simulink model "target_model"  (R2019a)
settings: Solver=FixedStepDiscrete  StartTime=0.0  StopTime=inf  RelTol=1e-3  EnableMultiTasking=on
PreLoadFcn:
  | load('visionhdlLaneDetectionInit.mat');
  | 
  | %Birds-Eye View Parameters:
  | T_unreal = [-0.346719845290643,-3.45626583672944e-16,-2.42608110520569e-19;-1.76272742794994,-2.62399506819665,-0.00185184300876343;1283.14845282490,1569.57420684550,1];
  | shiftleft = single([-5,-5,-5,-5,-5,-5,-5,-5,-5,-5,   -5,-4,-2,-2,-2,-2,0,0,0,1,    1,2,3,4,5,6,7,10,11,13,     15,17,20,22,26,30,33,38,42,46]);
  | shiftright = single([-20,-20,-20,-20,-20,-20,-20,-20,-20,-20,    -20,-20,-20,-21,-22,-23,-24,-24,-24,-25,    -26,-27,-28,-29,-30,-32,-33,-35,-37,-39,    -41,-45,-46,-50,-53,-57,-61,-67,-72,-78]);
StartFcn:
  | warning('off','Coder:MATLAB:polyfit_RepeatedPointsOrRescale');
  | warning('off','Coder:MATLAB:rankDeficientMatrix');
StopFcn:
  | warning('on','Coder:MATLAB:polyfit_RepeatedPointsOrRescale');
  | warning('on','Coder:MATLAB:rankDeficientMatrix');
undefined symbols (not defined in the file): FPGALaneDetection, IO333, LaneDetectionFPGA_final, msgfpgachecks, SFP
libraries: speedgoatlib_hdlCoder_IO333 x8, xpcutilitieslib x3, visiongeotforms x3, simulink x2, visiontextngfix x2, xpcvideoutillib x2, speedgoatlib_hdlCoder_IO333_vision x1, xpcrtudplib x1
Description:
  | Lane Detection
  | Detect lanes from streaming video.
settings Model: Creator=The MathWorks, Inc.  LastModifiedBy=timo.straessle
settings SolverCC: ConcurrentTasks=on  AutoInsertRateTranBlk=on
settings DataIOCC: SaveFormat=StructureWithTime  SaveOutput=off  SaveTime=off  ReturnWorkspaceOutputs=off
settings OptimizationCC: BlockReduction=off  ConditionallyExecuteInputs=off  DefaultParameterBehavior=Inlined  OptimizeBlockIOStorage=off  BufferReuse=off  GlobalBufferReuse=off  ExpressionFolding=off  LocalBlockOutputs=off  EfficientMapNaN2IntZero=off  OptimizeDataStoreBuffers=off  BusAssignmentInplaceUpdate=off
settings DebuggingCC: AlgebraicLoopMsg=error  SingleTaskRateTransMsg=error  ParameterPrecisionLossMsg=none  StrictBusMsg=ErrorOnBusTreatedAsVector  ArithmeticOperatorsInVariantConditions=warning
settings HardwareCC: ProdBitPerPointer=32  ProdBitPerSizeT=32  ProdBitPerPtrDiffT=32  ProdLargestAtomicFloat=None  ProdWordSize=32  ProdLongLongMode=on  ProdHWDeviceType=Generic->32-bit x86 compatible  TargetBitPerPointer=64  TargetBitPerSizeT=64  TargetBitPerPtrDiffT=64  TargetLongLongMode=on  TargetIntDivRoundTo=Zero  TargetEndianess=LittleEndian  TargetWordSize=64  TargetHWDeviceType=MATLAB Host
settings SFSimCC: SimUseLocalCustomCode=off
settings RTWCC: SystemTargetFile=slrt.tlc  TLCOptions=-axpcCPUClockPoll=0  TemplateMakefile=slrt_default_tmf  Description=Simulink Real-Time  CodeExecutionProfiling=on  RTWCompilerOptimization=on
settings CodeAppCC: MaxIdLength=128
settings SimulinkRealTimeCC: SupportVariableSizeSignals=on  PreserveStateflowLocalDataDimensions=off  RL32LogTETModifier=off  xPCisModelTimeout=off  xPCModelTimeoutSecs=60  xPCConcurrentTasks=on
settings ConfigComp: CovMetricSettings=dsw  CovHtmlReporting=on  CovSaveCumulativeToWorkspaceVar=on  CovSaveSingleToWorkspaceVar=on  CovShowResultsExplorer=off  CovExternalEMLEnable=off

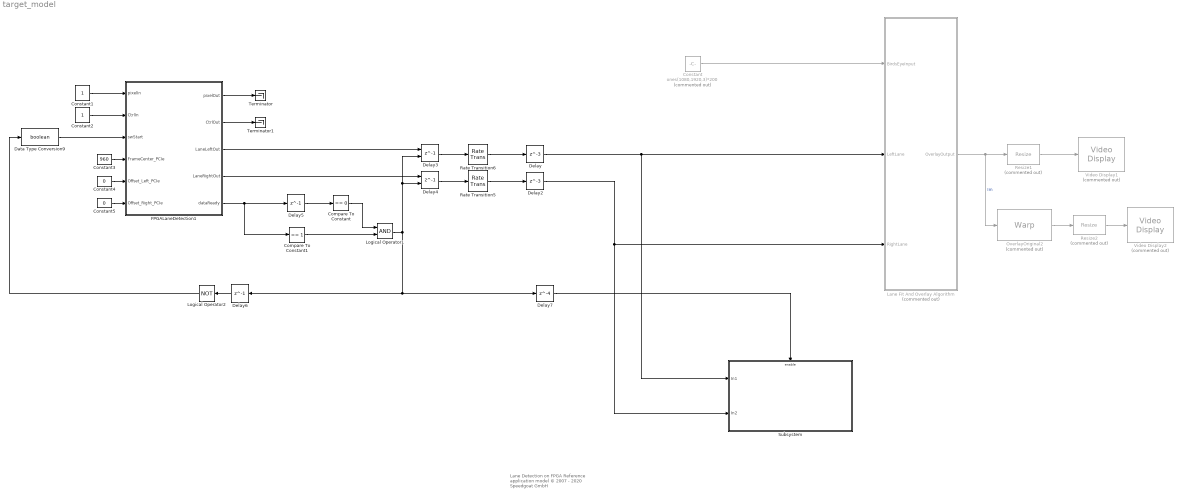
== system target_model ==
  note: Lane Detection on FPGA
      |
      | Reference application model
      | © 2007 - 2020 Speedgoat GmbH
  Compare To Constant : simulink/Logic and Bit Operations/Compare To Constant  relop===  const=0  OutDataTypeStr=boolean
  Compare To Constant1 : simulink/Logic and Bit Operations/Compare To Constant  relop===  const=1  OutDataTypeStr=boolean
  Constant : Constant  Commented=on  Value=ones(1080,1920,3)*200  OutDataTypeStr=uint8
  Constant1 : Constant
  Constant2 : Constant
  Constant3 : Constant  Value=960  OutDataTypeStr=fixdt(1,12,2^0,0)  SampleTime=-1
  Constant4 : Constant  Value=0  OutDataTypeStr=Inherit: Inherit via back propagation  SampleTime=-1
  Constant5 : Constant  Value=0  OutDataTypeStr=Inherit: Inherit via back propagation  SampleTime=-1
  Data Type Conversion9 : DataTypeConversion  OutDataTypeStr=boolean
  Delay : Delay  DelayLength=3
  Delay2 : Delay  DelayLength=3
  Delay3 : Delay  DelayLength=1  ShowEnablePort=on
      settings: InputPortMap=u0,e6
  Delay4 : Delay  DelayLength=1  ShowEnablePort=on
      settings: InputPortMap=u0,e6
  Delay5 : Delay  DelayLength=1
  Delay6 : Delay  DelayLength=1
  Delay7 : Delay  DelayLength=4
  FPGALaneDetection1 : Subsystem  InitFcn=msgfpgachecks;  mask(Speedgoat IO333-325k-SFP Interface Block){deviceIdx=0, slot=-1, ts=-1}
      mask prompts: deviceIdx "Device index:"; slot "PCI slot (-1: autosearch):"; ts "Sample time:"
      mask help: Simulink Real-Time Interface Block for Speedgoat IO333-325k-SFP.
      mask init:
      | mfpgaparameters;
      | TS = sg_hdlCoder_timestamp2DUTmask();
      mask Help: eval('speedgoatdoc_hdlc')
      mask Display: disp(sprintf('Speedgoat IO333-325k-SFP\nFPGA I/O Module\n\nTimestamp\n%s\n\nReference Design\nVersion 1.1\n\nMatlab R2019a\n\nPCIe Link Width: X4\nAurora Line Rate: 3.125\nAurora Byteswap: true\n', TS))
  Lane Fit And Overlay Algorithm : Subsystem  Commented=on
  Logical Operator1 : Logic  AllPortsSameDT=off  OutDataTypeStr=boolean
  Logical Operator2 : Logic  Operator=NOT  AllPortsSameDT=off  OutDataTypeStr=boolean
  OverlayOriginal2 : visiongeotforms/Warp  Commented=on  TransformMatrixSource=Custom  TransformMatrix=inv(T_unreal)  InterpolationMethod=Bilinear  BackgroundFillValue=0  OutputImagePositionSource=Custom  OutputImagePosition=[ 1, 1, 1920, 1080 ]  ROIInputPort=off  ROIValidityOutputPort=off  SimulateUsing=Code generation
      settings: SourceProductName=Computer Vision Toolbox  SourceProductBaseCode=VP
  Rate Transition5 : RateTransition  Deterministic=off  OutPortSampleTime=1/60
  Rate Transition6 : RateTransition  Deterministic=off  OutPortSampleTime=1/60
  Resize1 : visiongeotforms/Resize  Commented=on  specify=Output size as a percentage of input size  rfactor=[25 25]  outCols=25  outRows=25  outRowsCols=[25 35]  interp_method=Bilinear  antialias=on  useROI=off  roiFlag=off  roundingMode=Nearest  overflowMode=on  prodOutputMode=Binary point scaling  prodOutputWordLength=32  prodOutputFracLength=10  prodOutputSlope=2^-10  accumSlope=2^-10  outputSlope=2^-10
      settings: SourceProductName=Computer Vision Toolbox  SourceProductBaseCode=VP
  Resize2 : visiongeotforms/Resize  Commented=on  specify=Output size as a percentage of input size  rfactor=[25 25]  outCols=25  outRows=25  outRowsCols=[25 35]  interp_method=Bilinear  antialias=on  useROI=off  roiFlag=off  roundingMode=Nearest  overflowMode=on  prodOutputMode=Binary point scaling  prodOutputWordLength=32  prodOutputFracLength=10  prodOutputSlope=2^-10  accumSlope=2^-10  outputSlope=2^-10
      settings: SourceProductName=Computer Vision Toolbox  SourceProductBaseCode=VP
  Subsystem : Subsystem
  Terminator : Terminator
  Terminator1 : Terminator
  Video Display1 : xpcvideoutillib/Video Display  Commented=on  imagesignal=Single multidimensional signal  colorspace=RGB  vindex=1  showpreview=on
      settings: SourceProductName=Simulink Real-Time  SourceProductBaseCode=XP
  Video Display2 : xpcvideoutillib/Video Display  Commented=on  imagesignal=Single multidimensional signal  colorspace=RGB  vindex=2  showpreview=on
      settings: SourceProductName=Simulink Real-Time  SourceProductBaseCode=XP
  wires:
  Constant5/1 -> FPGALaneDetection1/6(Offset_Right_PCIe)
  Constant4/1 -> FPGALaneDetection1/5(Offset_Left_PCIe)
  Constant3/1 -> FPGALaneDetection1/4(FrameCenter_PCIe)
  Delay7/1 -> Subsystem/Enable
  Rate Transition6/1 -> Delay/1
  OverlayOriginal2/1 -> Resize2/1
  Delay2/1 -> Subsystem/2(In2), Lane Fit And Overlay Algorithm/3(RightLane)
  Delay4/1 -> Rate Transition5/1
  Rate Transition5/1 -> Delay2/1
  Compare To Constant1/1 -> Logical Operator1/2
  FPGALaneDetection1/5(dataReady) -> Compare To Constant1/1, Delay5/1
  Compare To Constant/1 -> Logical Operator1/1
  Logical Operator1/1 -> Delay7/1, Delay6/1, Delay4/2, Delay3/2
  Constant1/1 -> FPGALaneDetection1/1(pixelIn)
  Constant2/1 -> FPGALaneDetection1/2(CtrlIn)
  Resize2/1 -> Video Display2/1
  FPGALaneDetection1/2(CtrlOut) -> Terminator1/1
  FPGALaneDetection1/1(pixelOut) -> Terminator/1
  Delay5/1 -> Compare To Constant/1
  Lane Fit And Overlay Algorithm/1(OverlayOutput) -> Resize1/1, OverlayOriginal2/1  "Im"
  Delay3/1 -> Rate Transition6/1
  Logical Operator2/1 -> Data Type Conversion9/1
  FPGALaneDetection1/3(LaneLeftOut) -> Delay3/1
  Resize1/1 -> Video Display1/1
  Delay6/1 -> Logical Operator2/1
  FPGALaneDetection1/4(LaneRightOut) -> Delay4/1
  Constant/1 -> Lane Fit And Overlay Algorithm/1(BirdsEyeInput)
  Data Type Conversion9/1 -> FPGALaneDetection1/3(swStart)
  Delay/1 -> Subsystem/1(In1), Lane Fit And Overlay Algorithm/2(LeftLane)

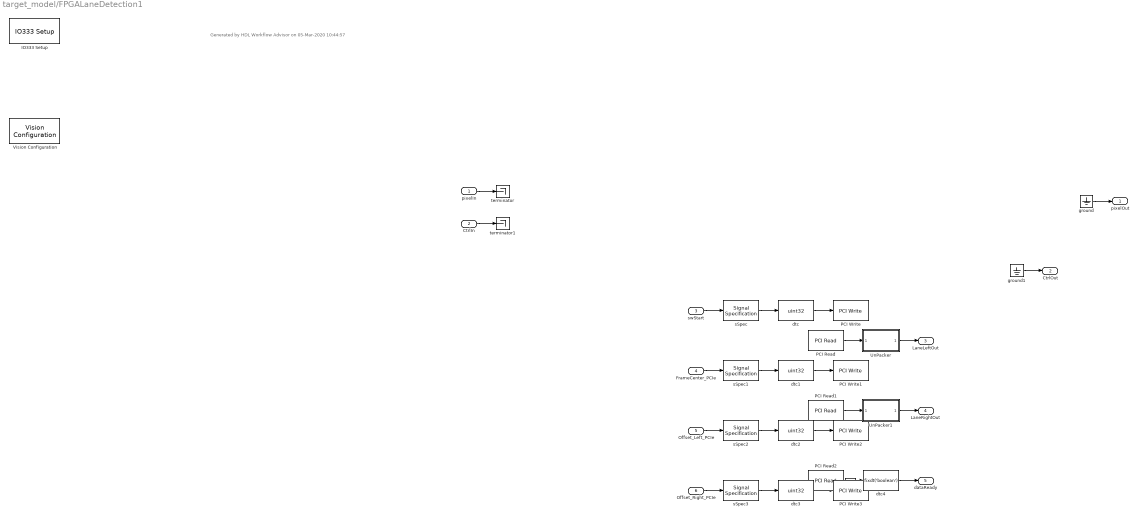
== system target_model/FPGALaneDetection1 ==
  note: Generated by HDL Workflow Advisor on 05-Mar-2020 10:44:57
  pixelIn : Inport
  CtrlIn : Inport  Port=2
  swStart : Inport  Port=3
  FrameCenter_PCIe : Inport  Port=4
  Offset_Left_PCIe : Inport  Port=5
  Offset_Right_PCIe : Inport  Port=6
  IO333 Setup : speedgoatlib_hdlCoder_IO333/IO333 Setup  mdl_ss_name=LaneDetectionFPGA_final/FPGALaneDetection  boardtype=IO333-325k-SFP  fpga_sync_mode=on  reset_mode=on  device_id=deviceIdx  pci_slot=slot  fpga_mat_file=E:\HDL_TMP\hdlsrc\LaneDetectionFPGA_final\FPGALaneDetection.mat  timestamp_mcs=05/03/20 10:41:08  timestamp=2003050958  tsreg=hex2dec('18')  bsf_file=FPGALaneDetection_2003050958.mcs  mcs=0
      settings: SourceProductName=Simulink Real-Time: Speedgoat HDL Coder Driver Library
  PCI Read : speedgoatlib_hdlCoder_IO333/PCI Read  device_id=deviceIdx  port_name=LaneLeftOut  port_offset=hex2dec('280')  port_type=uint32  port_dim=20  strobe=hex2dec('300')  sample_time=ts
      settings: SourceProductName=Simulink Real-Time: Speedgoat HDL Coder Driver Library
  PCI Read1 : speedgoatlib_hdlCoder_IO333/PCI Read  device_id=deviceIdx  port_name=LaneRightOut  port_offset=hex2dec('180')  port_type=uint32  port_dim=20  strobe=hex2dec('200')  sample_time=ts
      settings: SourceProductName=Simulink Real-Time: Speedgoat HDL Coder Driver Library
  PCI Read2 : speedgoatlib_hdlCoder_IO333/PCI Read  device_id=deviceIdx  port_name=dataReady  port_offset=hex2dec('114')  port_type=uint32  port_dim=1  strobe=0  sample_time=ts
      settings: SourceProductName=Simulink Real-Time: Speedgoat HDL Coder Driver Library
  PCI Write : speedgoatlib_hdlCoder_IO333/PCI Write  device_id=deviceIdx  port_name=swStart  port_offset=hex2dec('100')  port_type=uint32  port_dim=1  strobe=0  sample_time=ts
      settings: SourceProductName=Simulink Real-Time: Speedgoat HDL Coder Driver Library
  PCI Write1 : speedgoatlib_hdlCoder_IO333/PCI Write  device_id=deviceIdx  port_name=FrameCenter_PCIe  port_offset=hex2dec('104')  port_type=uint32  port_dim=1  strobe=0  sample_time=ts
      settings: SourceProductName=Simulink Real-Time: Speedgoat HDL Coder Driver Library
  PCI Write2 : speedgoatlib_hdlCoder_IO333/PCI Write  device_id=deviceIdx  port_name=Offset_Left_PCIe  port_offset=hex2dec('108')  port_type=uint32  port_dim=1  strobe=0  sample_time=ts
      settings: SourceProductName=Simulink Real-Time: Speedgoat HDL Coder Driver Library
  PCI Write3 : speedgoatlib_hdlCoder_IO333/PCI Write  device_id=deviceIdx  port_name=Offset_Right_PCIe  port_offset=hex2dec('10C')  port_type=uint32  port_dim=1  strobe=0  sample_time=ts
      settings: SourceProductName=Simulink Real-Time: Speedgoat HDL Coder Driver Library
  UnPacker : Subsystem
  UnPacker1 : Subsystem
  Vision Configuration : speedgoatlib_hdlCoder_IO333_vision/Vision Configuration  device_id=deviceIdx
  dtc{,1..3} (4 alike) : DataTypeConversion  OutDataTypeStr=uint32  ConvertRealWorld=Stored Integer (SI)  RndMeth=Zero
  dtc4 : DataTypeConversion  OutDataTypeStr=fixdt('boolean')  ConvertRealWorld=Stored Integer (SI)  RndMeth=Zero
  ground : Ground
  ground1 : Ground
  sSpec : SignalSpecification  OutDataTypeStr=fixdt('boolean')
  sSpec1 : SignalSpecification  OutDataTypeStr=fixdt(1,12,0)
  sSpec2 : SignalSpecification  OutDataTypeStr=fixdt(1,32,18)
  sSpec3 : SignalSpecification  OutDataTypeStr=fixdt(1,32,18)
  terminator : Terminator
  terminator1 : Terminator
  pixelOut : Outport
  CtrlOut : Outport  Port=2
  LaneLeftOut : Outport  Port=3
  LaneRightOut : Outport  Port=4
  dataReady : Outport  Port=5
  wires:
  pixelIn/1 -> terminator/1
  CtrlIn/1 -> terminator1/1
  swStart/1 -> sSpec/1
  sSpec/1 -> dtc/1
  dtc/1 -> PCI Write/1
  FrameCenter_PCIe/1 -> sSpec1/1
  sSpec1/1 -> dtc1/1
  dtc1/1 -> PCI Write1/1
  Offset_Left_PCIe/1 -> sSpec2/1
  sSpec2/1 -> dtc2/1
  dtc2/1 -> PCI Write2/1
  Offset_Right_PCIe/1 -> sSpec3/1
  sSpec3/1 -> dtc3/1
  dtc3/1 -> PCI Write3/1
  ground/1 -> pixelOut/1
  ground1/1 -> CtrlOut/1
  UnPacker/1(unpacked) -> LaneLeftOut/1
  PCI Read/1 -> UnPacker/1(packed)
  UnPacker1/1(unpacked) -> LaneRightOut/1
  PCI Read1/1 -> UnPacker1/1(packed)
  dtc4/1 -> dataReady/1
  PCI Read2/1 -> dtc4/1

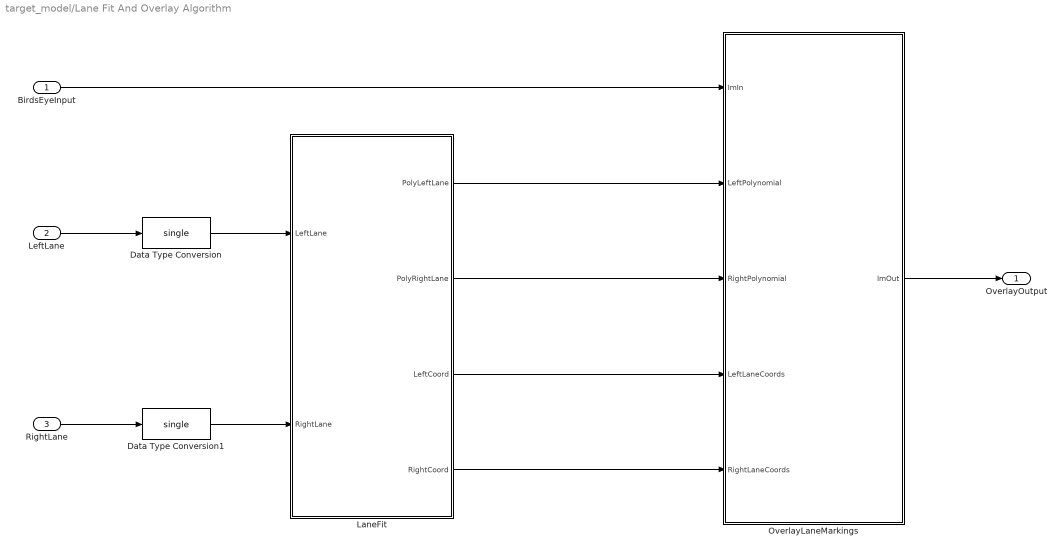
== system target_model/Lane Fit And Overlay Algorithm ==
  BirdsEyeInput : Inport
  LeftLane : Inport  Port=2
  RightLane : Inport  Port=3
  Data Type Conversion : DataTypeConversion  OutDataTypeStr=single
  Data Type Conversion1 : DataTypeConversion  OutDataTypeStr=single
  LaneFit : Subsystem
  OverlayLaneMarkings : Subsystem
  OverlayOutput : Outport
  wires:
  OverlayLaneMarkings/1(ImOut) -> OverlayOutput/1
  LaneFit/1(PolyLeftLane) -> OverlayLaneMarkings/2(LeftPolynomial)
  LaneFit/2(PolyRightLane) -> OverlayLaneMarkings/3(RightPolynomial)
  LeftLane/1 -> Data Type Conversion/1
  RightLane/1 -> Data Type Conversion1/1
  BirdsEyeInput/1 -> OverlayLaneMarkings/1(ImIn)
  LaneFit/3(LeftCoord) -> OverlayLaneMarkings/4(LeftLaneCoords)
  LaneFit/4(RightCoord) -> OverlayLaneMarkings/5(RightLaneCoords)
  Data Type Conversion/1 -> LaneFit/1(LeftLane)
  Data Type Conversion1/1 -> LaneFit/2(RightLane)

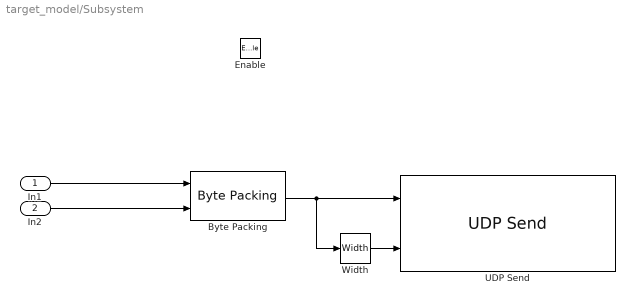
== system target_model/Subsystem ==
  In1 : Inport
  In2 : Inport  Port=2
  Enable : EnablePort
  "Byte Packing " : xpcutilitieslib/Byte Packing   MaskPackedDataType=uint8  MaskUnpackedDataTypes={['uint16'],['uint16']}  MaskAlignment=1
  UDP Send : xpcrtudplib/UDP Send  ipAddressVal=Use host-target connection  localPort=25001  toAddress=192.168.7.2  toPort=8001  sampleTime=-1
      settings: SourceProductName=Simulink Real-Time  SourceProductBaseCode=XP
  Width : Width
  wires:
  "Byte Packing "/1 -> UDP Send/1, Width/1
  In2/1 -> "Byte Packing "/2
  In1/1 -> "Byte Packing "/1
  Width/1 -> UDP Send/2

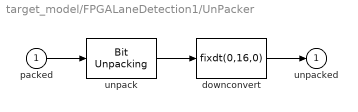
== system target_model/FPGALaneDetection1/UnPacker ==
  packed : Inport
  downconvert : DataTypeConversion  OutDataTypeStr=fixdt(0,16,0)  ConvertRealWorld=Stored Integer (SI)  RndMeth=Zero
  unpack : xpcutilitieslib/Bit Unpacking   SignExtend=on  MaskBitPatterns={[0:15 16:31 32:47 48:63 64:79 80:95 96:111 112:127 128:143 144:159 160:175 176:191 192:207 208:223 224:239 240:255 256:271 272:287 288:303 304:319 320:335 336:351 352:367 368:383 384:399 400:415 416:431 432:447 448:463 464:479 480:495 496:511 512:527 528:543 544:559 560:575 576:591 592:607 608:623 624:639 ]}  MaskPackDataType=uint32  MaskPackDataSize=20  MaskUnpackDataTypes={'uint16'}  MaskUnpackDataSizes={40}
      settings: SourceProductName=Simulink Real-Time  SourceProductBaseCode=XP
  unpacked : Outport
  wires:
  packed/1 -> unpack/1
  unpack/1 -> downconvert/1
  downconvert/1 -> unpacked/1

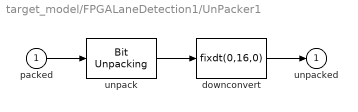
== system target_model/FPGALaneDetection1/UnPacker1 ==
  packed : Inport
  downconvert : DataTypeConversion  OutDataTypeStr=fixdt(0,16,0)  ConvertRealWorld=Stored Integer (SI)  RndMeth=Zero
  unpack : xpcutilitieslib/Bit Unpacking   SignExtend=on  MaskBitPatterns={[0:15 16:31 32:47 48:63 64:79 80:95 96:111 112:127 128:143 144:159 160:175 176:191 192:207 208:223 224:239 240:255 256:271 272:287 288:303 304:319 320:335 336:351 352:367 368:383 384:399 400:415 416:431 432:447 448:463 464:479 480:495 496:511 512:527 528:543 544:559 560:575 576:591 592:607 608:623 624:639 ]}  MaskPackDataType=uint32  MaskPackDataSize=20  MaskUnpackDataTypes={'uint16'}  MaskUnpackDataSizes={40}
      settings: SourceProductName=Simulink Real-Time  SourceProductBaseCode=XP
  unpacked : Outport
  wires:
  packed/1 -> unpack/1
  unpack/1 -> downconvert/1
  downconvert/1 -> unpacked/1

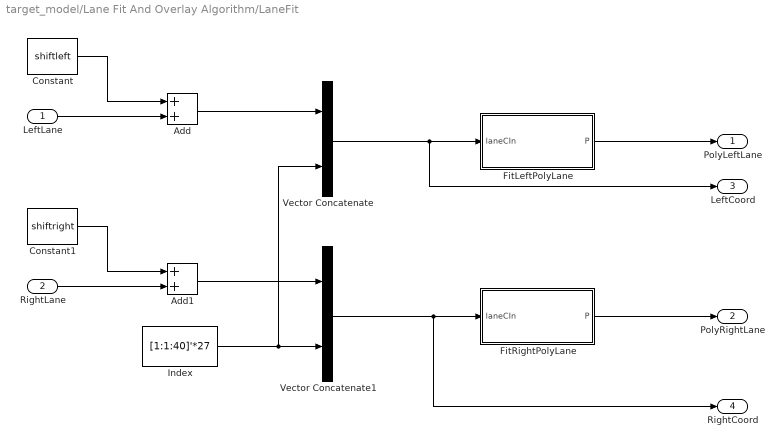
== system target_model/Lane Fit And Overlay Algorithm/LaneFit ==
  LeftLane : Inport
  RightLane : Inport  Port=2
  Add : Sum
  Add1 : Sum
  Constant : Constant  Value=shiftleft
  Constant1 : Constant  Value=shiftright
  FitLeftPolyLane : MATLAB Function  TreatAsAtomicUnit=on
  FitRightPolyLane : MATLAB Function  TreatAsAtomicUnit=on
  Index : Constant  Value=[1:1:40]'*27  VectorParams1D=off  OutDataTypeStr=single  SampleTime=-1
  Vector Concatenate : Concatenate  Mode=Multidimensional array  ConcatenateDimension=2
  Vector Concatenate1 : Concatenate  Mode=Multidimensional array  ConcatenateDimension=2
  PolyLeftLane : Outport
  PolyRightLane : Outport  Port=2
  LeftCoord : Outport  Port=3
  RightCoord : Outport  Port=4
  wires:
  FitLeftPolyLane/1(P) -> PolyLeftLane/1
  Vector Concatenate/1 -> FitLeftPolyLane/1(laneCIn), LeftCoord/1
  Index/1 -> Vector Concatenate/2, Vector Concatenate1/2
  Vector Concatenate1/1 -> FitRightPolyLane/1(laneCIn), RightCoord/1
  FitRightPolyLane/1(P) -> PolyRightLane/1
  LeftLane/1 -> Add/2
  RightLane/1 -> Add1/2
  Constant/1 -> Add/1
  Add/1 -> Vector Concatenate/1
  Constant1/1 -> Add1/1
  Add1/1 -> Vector Concatenate1/1

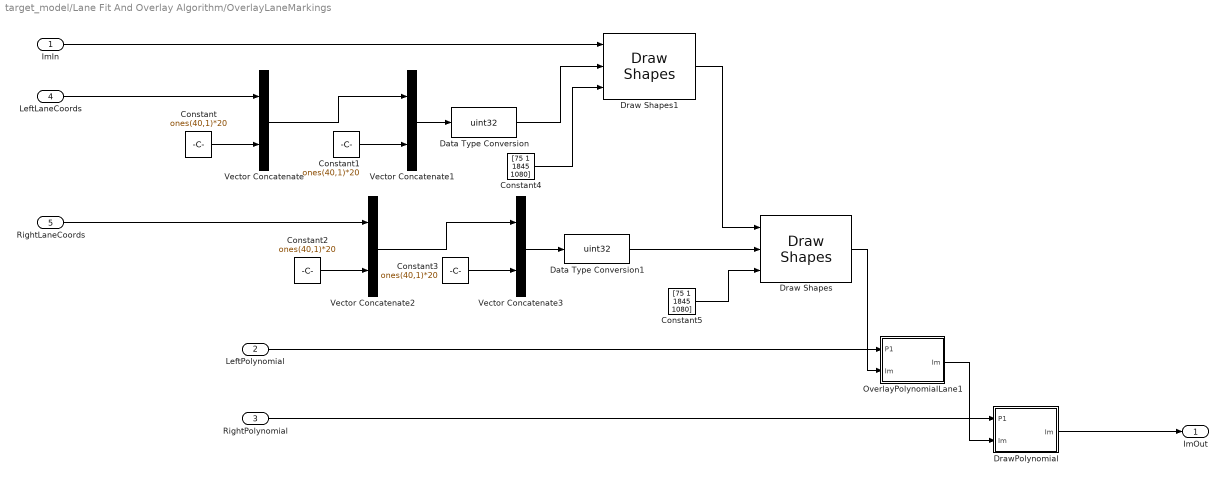
== system target_model/Lane Fit And Overlay Algorithm/OverlayLaneMarkings ==
  ImIn : Inport
  LeftPolynomial : Inport  Port=2
  RightPolynomial : Inport  Port=3
  LeftLaneCoords : Inport  Port=4
  RightLaneCoords : Inport  Port=5
  Constant{,1..3} (4 alike) : Constant  Value=ones(40,1)*20  OutDataTypeStr=single  SampleTime=-1
  Constant4 : Constant  Value=[75 1 1845 1080]  OutDataTypeStr=uint32  SampleTime=-1
  Constant5 : Constant  Value=[75 1 1845 1080]  OutDataTypeStr=uint32  SampleTime=-1
  Data Type Conversion : DataTypeConversion  OutDataTypeStr=uint32
  Data Type Conversion1 : DataTypeConversion  OutDataTypeStr=uint32
  Draw Shapes : visiontextngfix/Draw Shapes  shape=Rectangles  fill=off  lineWidth=4  fillClrSource=Specify via dialog  display=User-specified value  intensity=200  color=[83, 219, 192]  opacity=0.6  viewport=Specify region of interest via port  antialiasing=off  inType=Obsolete  imagePorts=One multidimensional signal  roundingMode=Floor  overflowMode=off  memoryMode=Specify word length  memoryWordLength=16  prodOutputMode=Binary point scaling  prodOutputWordLength=32  prodOutputFracLength=14  prodOutputSlope=2^-14  accumSlope=2^-14  memoryFracLength=15
      settings: SourceProductName=Computer Vision Toolbox
  Draw Shapes1 : visiontextngfix/Draw Shapes  shape=Rectangles  fill=off  lineWidth=4  fillClrSource=Specify via dialog  display=User-specified value  intensity=200  color=[255, 26,0]  opacity=0.6  viewport=Specify region of interest via port  antialiasing=off  inType=Obsolete  imagePorts=One multidimensional signal  roundingMode=Floor  overflowMode=off  memoryMode=Specify word length  memoryWordLength=16  prodOutputMode=Binary point scaling  prodOutputWordLength=32  prodOutputFracLength=14  prodOutputSlope=2^-14  accumSlope=2^-14  memoryFracLength=15
      settings: SourceProductName=Computer Vision Toolbox
  DrawPolynomial : MATLAB Function  TreatAsAtomicUnit=on
  OverlayPolynomialLane1 : MATLAB Function  TreatAsAtomicUnit=on
  Vector Concatenate{,1..3} (4 alike) : Concatenate  Mode=Multidimensional array  ConcatenateDimension=2
  ImOut : Outport
  wires:
  Vector Concatenate/1 -> Vector Concatenate1/1
  Draw Shapes/1 -> OverlayPolynomialLane1/2("Im ")
  OverlayPolynomialLane1/1(Im) -> DrawPolynomial/2("Im ")
  RightLaneCoords/1 -> Vector Concatenate2/1
  ImIn/1 -> Draw Shapes1/1
  Vector Concatenate1/1 -> Data Type Conversion/1
  Constant/1 -> Vector Concatenate/2
  DrawPolynomial/1(Im) -> ImOut/1
  LeftLaneCoords/1 -> Vector Concatenate/1
  Constant1/1 -> Vector Concatenate1/2
  LeftPolynomial/1 -> OverlayPolynomialLane1/1(P1)
  Vector Concatenate3/1 -> Data Type Conversion1/1
  Constant3/1 -> Vector Concatenate3/2
  Constant4/1 -> Draw Shapes1/3
  RightPolynomial/1 -> DrawPolynomial/1(P1)
  Vector Concatenate2/1 -> Vector Concatenate3/1
  Data Type Conversion1/1 -> Draw Shapes/2
  Draw Shapes1/1 -> Draw Shapes/1
  Constant5/1 -> Draw Shapes/3
  Data Type Conversion/1 -> Draw Shapes1/2
  Constant2/1 -> Vector Concatenate2/2

== matlab function target_model/Lane Fit And Overlay Algorithm/LaneFit/FitLeftPolyLane ==
  data: laneCIn input; P output
function P  = fitLane(laneCIn)

%#codegen

persistent P1;
if isempty(P1)
    P1 = [0 0 0];
end

leftLimit = 50;

% laneC = zeros(40,2);
inliersMask = zeros(1,100);
inlierTable1 = zeros(2,100);
P1T= single([0 0 0]);
% % aviod using sortrows (time complexity O(nlogn))
% % now O(n) oeprations
laneC = single(zeros(40,2));
 numG = 0;
 for jj = 1:1:40
     if(laneCIn(jj,1)>leftLimit)
         numG = numG+1;
         laneC(numG,1:2) = single(laneCIn(jj,1:2));
     end
 end


% ignore when inliers/total < curInliersRatio
curInliersRatio = 0.4;

% inlierIndex1-1 = num of inliers in best model
% is also used to determine whether a best model is found
inlierIndex1 = 0;

% K = log(1-P)/log(1-w^s)
K = 70; % max iteration

distanceMax = 60; % distance Threshold

curvatureMax = 0.003; % curvature Threshold for P(1); maybe removed for curved lanes


if numG>3
    
    %%% Use RANSAC for robust fit of 2nd order polynomial
    
    for ii = 1:1:K

        a = randperm(numG,3);
        
        P1T = polyfit(laneC(a,1), laneC(a,1),2);
        
        % O(n) operations
        numInliers = 0;
        for jj = 1:1:numG
            x1 = floor(polyval(P1T,laneC(jj,1)));
            inliersMask(jj) = abs(x1-laneC(jj,1))<distanceMax;
            if(inliersMask(jj))
                numInliers = numInliers + 1;
            end
        end

        if ((numInliers/numG)>curInliersRatio && abs(P1T(1))<curvatureMax && numInliers>2)
            % record the inliers for current best model  
            curInliersRatio = numInliers/numG;
            inlierIndex1 = 1;
            for jj = 1:1:numG
                if(inliersMask(jj))
                    inlierTable1(1,inlierIndex1) = laneC(jj,2);
                    inlierTable1(2,inlierIndex1) = laneC(jj,1);
                    inlierIndex1 = inlierIndex1 + 1;
                end
            end
        end
        
    end
  
end

    P1T = polyfit(inlierTable1(1,1:inlierIndex1-1), inlierTable1(2,1:inlierIndex1-1),2);


if abs(P1T(1))<curvatureMax % if found a best model; initial inlierIndex1 = 0;
    % refine the fitted line using all inliers
    P1 = P1T;
end

P = P1;

== matlab function target_model/Lane Fit And Overlay Algorithm/LaneFit/FitRightPolyLane ==
  data: laneCIn input; P output
function P  = fitLane(laneCIn)

%#codegen

persistent P1;
if isempty(P1)
    P1 = [0 0 0];
end

leftLimit = 50;

% laneC = zeros(40,2);
inliersMask = zeros(1,100);
inlierTable1 = zeros(2,100);
P1T= single([0 0 0]);
% % aviod using sortrows (time complexity O(nlogn))
% % now O(n) oeprations
laneC = single(zeros(40,2));
 numG = 0;
 for jj = 1:1:40
     if(laneCIn(jj,1)>leftLimit)
         numG = numG+1;
         laneC(numG,1:2) = single(laneCIn(jj,1:2));
     end
 end


% ignore when inliers/total < curInliersRatio
curInliersRatio = 0.4;

% inlierIndex1-1 = num of inliers in best model
% is also used to determine whether a best model is found
inlierIndex1 = 0;

% K = log(1-P)/log(1-w^s)
K = 70; % max iteration

distanceMax = 60; % distance Threshold

curvatureMax = 0.003; % curvature Threshold for P(1); maybe removed for curved lanes


if numG>3
    
    %%% Use RANSAC for robust fit of 2nd order polynomial
    
    for ii = 1:1:K

        a = randperm(numG,3);
        
        P1T = polyfit(laneC(a,1), laneC(a,1),2);
        
        % O(n) operations
        numInliers = 0;
        for jj = 1:1:numG
            x1 = floor(polyval(P1T,laneC(jj,1)));
            inliersMask(jj) = abs(x1-laneC(jj,1))<distanceMax;
            if(inliersMask(jj))
                numInliers = numInliers + 1;
            end
        end

        if ((numInliers/numG)>curInliersRatio && abs(P1T(1))<curvatureMax && numInliers>2)
            % record the inliers for current best model  
            curInliersRatio = numInliers/numG;
            inlierIndex1 = 1;
            for jj = 1:1:numG
                if(inliersMask(jj))
                    inlierTable1(1,inlierIndex1) = laneC(jj,2);
                    inlierTable1(2,inlierIndex1) = laneC(jj,1);
                    inlierIndex1 = inlierIndex1 + 1;
                end
            end
        end
        
    end
  
end

    P1T = polyfit(inlierTable1(1,1:inlierIndex1-1), inlierTable1(2,1:inlierIndex1-1),2);


if abs(P1T(1))<curvatureMax % if found a best model; initial inlierIndex1 = 0;
    % refine the fitted line using all inliers
    P1 = P1T;
end

P = P1;

== matlab function target_model/Lane Fit And Overlay Algorithm/OverlayLaneMarkings/DrawPolynomial ==
  data: P1 input; Im output; Im input
function Im  = DrawLane(P1,Im)
%#codegen

% ipmImage = uint8(zeros(900,640,3));
% HD: uint8(zeros(1575,1440,3));
RGBVal = [0,255,9];



  for ii = 1:1:1080
      x1E = floor(polyval(P1,ii));
      
      if x1E <=5 || isnan(x1E)
          x1E = 6;
      elseif x1E>=1919
          x1E=1919;
      end
      
 
      Im(ii,x1E+0,:) = RGBVal;
      Im(ii,x1E-1,:) = RGBVal;
      Im(ii,x1E-2,:) = RGBVal;
      Im(ii,x1E-3,:) = RGBVal;
      Im(ii,x1E-4,:) = RGBVal;
      Im(ii,x1E-5,:) = RGBVal;

      
      
  end


% Im = ipmImage;

== matlab function target_model/Lane Fit And Overlay Algorithm/OverlayLaneMarkings/OverlayPolynomialLane1 ==
  data: P1 input; Im output; Im input
function Im  = fcn(P1,Im)
%#codegen

% ipmImage = uint8(zeros(900,640,3));
% HD: uint8(zeros(1575,1440,3));
RGBVal = [0,255,9];



  for ii = 1:1:1080
      x1E = floor(polyval(P1,ii));
      
      if x1E <=50 || isnan(x1E)
          x1E = 6;
      elseif x1E>=1919
          x1E=1919;
      end
      
 
      Im(ii,x1E+0,:) = RGBVal;
      Im(ii,x1E-1,:) = RGBVal;
      Im(ii,x1E-2,:) = RGBVal;
      Im(ii,x1E-3,:) = RGBVal;
      Im(ii,x1E-4,:) = RGBVal;
      Im(ii,x1E-5,:) = RGBVal;

      
      
  end


% Im = ipmImage;
